simulink model "sm_suspension_templates"  (R2021b)
settings: Solver=ode15s  StartTime=0.0  StopTime=60  MaxStep=0.01  RelTol=1e-3  EnableMultiTasking=on
model workspace: external: MATLAB File sm_suspension_templates_params.m (data not in the file)
undefined symbols (not defined in the file or in its folder): dwb, mp, platform, pr, sm_suspension_templates_roadgen, wheel, X, Y, Z
libraries: sm_lib x108, sm_suspension_templates_lib x60, nesl_utility x7
(part 1 of 7)
CloseFcn:
  | clear simlog_sm_suspension_templates
Description:
  | Independent Suspension System Templates
settings Model: Creator=The MathWorks, Inc.  LastModifiedBy=The MathWorks, Inc.
settings SolverCC: AlgebraicLoopSolver=TrustRegion
settings DataIOCC: SaveFormat=Array  SaveOutput=off  ReturnWorkspaceOutputs=off
settings OptimizationCC: ExpressionDepthLimit=2147483647  LifeSpan=inf
settings DebuggingCC: UnderspecifiedInitializationDetection=Classic  MergeDetectMultiDrivingBlocksExec=none  AllowSymbolicDim=off  StateNameClashWarn=warning  SFUnexpectedBacktrackingDiag=warning  SFNoUnconditionalDefaultTransitionDiag=warning  SFExecutionAtInitializationDiag=none  SFMachineParentedDataDiag=warning  ArithmeticOperatorsInVariantConditions=warning
settings HardwareCC: ProdBitPerPointer=32  ProdBitPerSizeT=32  ProdBitPerPtrDiffT=32  ProdLargestAtomicFloat=None  ProdIntDivRoundTo=Undefined  ProdEndianess=Unspecified  ProdWordSize=32  ProdHWDeviceType=32-bit Generic
settings ModelReferenceCC: PropagateSignalLabelsOutOfModel=off
settings SFSimCC: SimUseLocalCustomCode=off  CustomCodeUndefinedFunction=UseInterfaceOnly
settings RTWCC: RTWUseLocalCustomCode=off
settings CodeAppCC: StateflowObjectComments=on
settings GRTTargetCC: TargetLangStandard=C89/C90 (ANSI)
settings ConfigComp: CovScope=ReferencedModels  CovIncludeTopModel=off  CovMetricSettings=dw  CovSaveCumulativeToWorkspaceVar=on  CovSaveSingleToWorkspaceVar=on  CovExternalEMLEnable=off  CovSFcnEnable=off
settings SimscapeCC: SimscapeNormalizeSystem=off  SimscapeNominalValues="[{\"value\":\"10\",\"unit\":\"V\"},{\"value\":\"1\",\"unit\":\"A\"},{\"value\":\"10\",\"unit\":\"N*m\"},{\"value\":\"10\",\"unit\":\"bar\"},{\"value\":\"100\",\"unit\":\"kJ/kg\"},{\"value\":\"1\",\"unit\":\"kW\"},{\"value\":\"300\",\"unit\":\"K\"},{\"value\":\"100\",\"unit\":\"cm^3/s\"},{\"value\":\"1\",\"unit\":\"kN\"},{\"value\":\"1\",\"unit\":\"g/cm^3\"},{\"value\":\"1\",\"unit\":\"l\"},{\"value\":\"1\",\"unit\":\"cm^2\"},{\"value\":\"60\",\"unit\":\"Hz\"}]"  SimscapeLogType=all  SimscapeLogSimulationStatistics=on  SimscapeLogName=simlog_sm_suspension_templates  SimscapeLogDataHistory=10000
settings ConfigurationSet: Description=SimMechanics 2G
settings DiagnosticsConfigSet: SimMechanicsUnconnectedFramePorts=none  SimMechanicsUnsatisfiedHighPriorityTargets=none
settings ExplorerConfigSet: InternalSimMechanicsExplorerSettings="<ExplorerConfiguration><canonicalview>default</canonicalview><AnimationSetting><BasePlaybackSpeed>1.0</BasePlaybackSpeed><PlaybackSpeedFactor>1.0</PlaybackSpeedFactor></AnimationSetting><TilePanel><TileInfo><Tiles Columns=\"1\" Count=\"1\" Rows=\"1\"><Column Left=\"2\" Weight=\"1\"/><Column Left=\"827\"/><Row Top=\"2\" Weight=\"1\"/><Row Top=\"666\"/><Tile Height=\"1\" Width=\"1\" X=\"0\" Y=\"0\"/></Tiles></TileInfo><SceneInfo><SceneViewer><BGColor><R>0.60000002384185791</R><G>0.60000002384185791</G><B>0.60000002384185791</B></BGColor><Camera><Position><X>0</X><Y>-4.48140033882927202</Y><Z>0.554502487182617188</Z></Position><Center><X>0</X><Y>-0.245328903198242188</Y><Z>0.554502487182617188</Z></Center><Up><X>0</X><Y>-0</Y><Z>1</Z></Up><Left>-1.15500002503395094</Left><Right>1.15500002503395094</Right><Bottom>-0.792227599024772688</Bottom><Top>0.792227599024772688</Top></Camera></SceneViewer></SceneInfo></TilePanel></ExplorerConfiguration>"

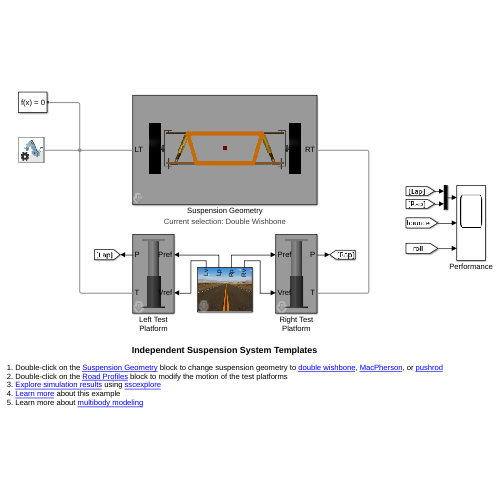
[thumbnail: Simulink's stored preview of the top-level diagram]
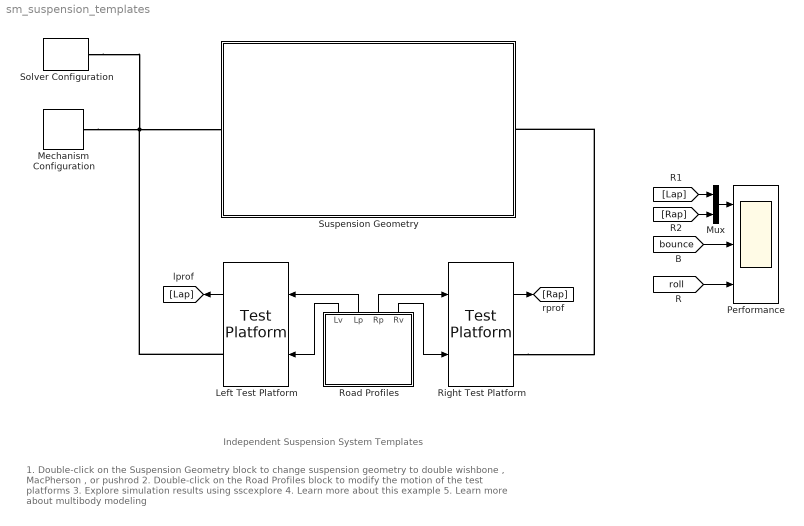
== system sm_suspension_templates ==
  note: Independent Suspension System Templates
  note: 1. Double-click on the Suspension Geometry block to change suspension geometry to double wishbone , MacPherson , or pushrod
      | 2. Double-click on the Road Profiles block to modify the motion of the test platforms
      | 3. Explore simulation results using sscexplore
      | 4. Learn more about this example
      | 5. Learn more about multibody modeling
  Left Test Platform : sm_suspension_templates_lib/Test Platform  Ro=platform.cylinder.outerradius  Ri=platform.cylinder.innerradius  Rf=platform.cylinder.flangeradius  Tf=platform.cylinder.flangethickness  Hc=platform.cylinder.height  cclr=platform.cylinder.color  loc=platform.cylinder.leftlocation  Rip=platform.piston.innerradius  Hp=platform.piston.height  pclr=platform.piston.color  L=platform.base.length  W=platform.base.width  H=platform.base.thickness  clr=platform.base.color  Kp=platform.controller.k  Kd=platform.controller.kd  rho=platform.density
      settings: SourceProductBaseCode=MS
  Mechanism Configuration : sm_lib/Utilities/Mechanism Configuration  UniformGravity=Constant  GravityVector=[0 0 -9.80665]  GravityUnits=m/s^2  LinearizationDelta=0.001  JointModeTransitionNonlinearIterations=2
  Mux : Mux  Inputs=2
  Performance : Scope  NumInputPorts=3
  Right Test Platform : sm_suspension_templates_lib/Test Platform  Ro=platform.cylinder.outerradius  Ri=platform.cylinder.innerradius  Rf=platform.cylinder.flangeradius  Tf=platform.cylinder.flangethickness  Hc=platform.cylinder.height  cclr=platform.cylinder.color  loc=platform.cylinder.rightlocation  Rip=platform.piston.innerradius  Hp=platform.piston.height  pclr=platform.piston.color  L=platform.base.length  W=platform.base.width  H=platform.base.thickness  clr=platform.base.color  Kp=platform.controller.k  Kd=platform.controller.kd  rho=platform.density
      settings: SourceProductBaseCode=MS
  Road Profiles : Subsystem  mask(Road Profile Generator){Ti=1, Ts=5.5, Tb=1, Fl=0.5, Al=5, Fm=3, Am=5, Fh=5, Ah=5, Ps=2, As=5, Wp=0.1, Pp=2, Ap=5, Ad=25}
      mask prompts: Ti "Start time (s):"; Ts "Duration of each segment (s):"; Tb "Buffer between segments (s):"; Fl "Frequency (Hz):"; Al "Amplitude (cm):"; Fm "Frequency (Hz):"; Am "Amplitude (cm):"; Fh "Frequency (Hz):"; Ah "Amplitude (cm):"; Ps "Period (s):"; As "Amplitude (cm):"; Wp "Width (s):"; Pp "Period (s):"; Ap "Amplitude (cm):"; Ad "Depth (cm):"
      mask help:
      | This block generates test road profiles for the left and right tires. A road profile is comprised of the following:
      |
      | 1  - Low frequency sinusoid with the left and right road profiles in phase
      | 2  - Low frequency sinusoid with the left and right road profiles out of phase
      | 3  - Mid frequency sinusoid with the left and right road profiles in phase
      | 4  - Mid frequency sinusoid with the left and right road profiles out of phase
      | 5  - High frequency sinusoid with the left and right road profiles in phase
      | 6  - High frequency sinusoid with the left and right road profiles out of phase
      | 7  - Step with the left and right road profiles in phase
      | 8  - Step with the left and right road profiles out of phase
      | 9  - Pulse with the left and right road profiles in phase
      | 10 - Pulse with the left and right road profiles out of phase
      | 11 - Large step down (dive)
      mask DialogControl ParameterTabVar0 Prompt: Time
      mask DialogControl ParameterTabVar01 Prompt: Low Freq
      mask DialogControl ParameterTabVar012 Prompt: Mid Freq
      mask DialogControl ParameterTabVar0123 Prompt: High Freq
      mask DialogControl ParameterTabVar01234 Prompt: Step
      mask DialogControl ParameterTabVar012345 Prompt: Pulse
      mask DialogControl ParameterTabVar0123456 Prompt: Dive
      mask Display:
      | image(imread(fullfile(matlabroot,...
      |     'toolbox','physmod','sm','smdemos',...
      |     'suspension_templates','images','sm_isuspension_road.png')));
  Solver Configuration : nesl_utility/Solver Configuration  PhysicalDomain=network_engine_domain  SubClassName=solver  LeftPortType=input  RightPortType=generic  Tones=[]  Harmonics=[]  SimulateNoise=off  Profile=off  UseLocalSampling=off  EnableSwitchedLinearOptims=on  FrequencyDomain=off  UseCCode=off  RelTol=0.001  AbsTol=1e-06  MinStep=1e-09  ToWorkspace=off  RevertToSquareIcSolve=off  NumHomotopyIterations=100  PhasorMode=off  PhasorModeNumHarmonics=1  DoDC=off  ResidualTolerance=1e-09  UseLocalSolver=off  LocalSolverChoice=NE_BACKWARD_EULER_ADVANCER  LocalSolverSampleTime=0.001  DoFixedCost=off  MaxNonlinIter=3  MaxModeIter=2  ComputeImpulses=off  ImpulseIterations=2  LinearAlgebra=Sparse  EquationFormulation=NE_TIME_EF  DelaysMemoryBudget=1024  AutomaticFiltering=on  FilteringTimeConstant=0.001  PartitionStorageMethod=AS_NEEDED  PartitionMemoryBudget=1024  PartitionMethod=FAST
      settings: SourceProductBaseCode=PW,SS
  Suspension Geometry : Subsystem  mask{SuspensionType=Double Wishbone}
      mask prompts: SuspensionType "Suspension Type:"
      mask init:
      | ST = get_param(gcb,'SuspensionType');
      | mdl = gcs;
      | switch ST
      |     case 'Double Wishbone'
      |         set_param([mdl,'/Suspension Geometry/Independent Suspension Geometry'],'OverrideUsingVariant','DoubleWishbone')
      |     case 'MacPherson'
      |         set_param([mdl,'/Suspension Geometry/Independent Suspension Geometry'],'OverrideUsingVariant','MacPherson')
      |     case 'Pushrod'
      |         set_param([mdl,'/Suspension Geometry/Independent Suspension Geometry'],'OverrideUsingVariant','Pushrod')
      | end
      settings: AttributesFormatString=Current selection: %<SuspensionType>
      mask TypeOptions SuspensionType: Double Wishbone | MacPherson | Pushrod
      mask Display:
      | ST = get_param(gcb,'SuspensionType');
      | switch ST
      |     case 'Double Wishbone'
      |         image(imread(fullfile(matlabroot,...
      |             'toolbox','physmod','sm','smdemos',...
      |             'suspension_templates','images','sm_isuspension_dwishboneassm.png')));
      |     case 'MacPherson'
      |         image(imread(fullfile(matlabroot,...
      |             'toolbox','physmod','sm','smdemos',...
      |             'suspension_templates','images','sm_isuspension_macphersonassm.png')));
      |     case 'Pushrod'
      |         image(imread(fullfile(matlabroot,...
      |             'toolbox','physmod','sm','smdemos',...
      |             'suspension_templates','images','sm_isuspension_pushrodassm.png')));
      | end
      | 
      | port_label('LConn',1,'LT');
      | port_label('RConn',1,'RT');
  wires:
  [bounce] -> Performance/2
  [roll] -> Performance/3
  [Lap] -> Mux/1
  [Rap] -> Mux/2
  Road Profiles/2(Lp) -> Left Test Platform/1
  Road Profiles/1(Lv) -> Left Test Platform/2
  Left Test Platform/1 -> [Lap]
  Right Test Platform/1 -> [Rap]
  Road Profiles/3(Rp) -> Right Test Platform/1
  Road Profiles/4(Rv) -> Right Test Platform/2
  Mux/1 -> Performance/1
  connections:
  Left Test Platform/RConn1 -- Suspension Geometry/LConn1 -- Solver Configuration/RConn1 -- Mechanism Configuration/RConn1
  Right Test Platform/RConn1 -- Suspension Geometry/RConn1

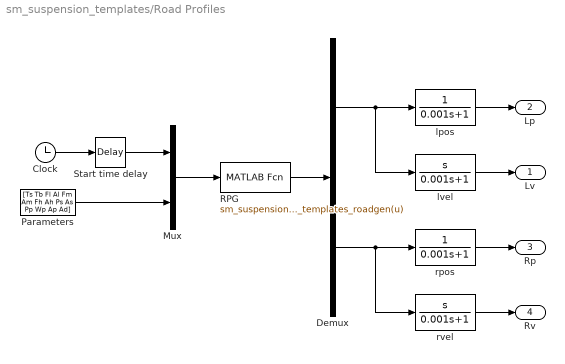
== system sm_suspension_templates/Road Profiles ==
  Clock : Clock
  Demux : Demux  Outputs=2
  Mux : Mux  Inputs=2
  Parameters : Constant  Value=[Ts Tb Fl Al Fm Am Fh Ah Ps As Pp Wp Ap Ad]
  RPG : MATLABFcn  MATLABFcn=sm_suspension_templates_roadgen(u)  Output1D=off
  Start time delay : TransportDelay  DelayTime=Ti  BufferSize=2048
  lpos : TransferFcn  Denominator=[0.001 1]
  lvel : TransferFcn  Numerator=[1 0]  Denominator=[0.001 1]
  rpos : TransferFcn  Denominator=[0.001 1]
  rvel : TransferFcn  Numerator=[1 0]  Denominator=[0.001 1]
  Lv : Outport  VectorParamsAs1DForOutWhenUnconnected=off
  Lp : Outport  Port=2  VectorParamsAs1DForOutWhenUnconnected=off
  Rp : Outport  Port=3  VectorParamsAs1DForOutWhenUnconnected=off
  Rv : Outport  Port=4  VectorParamsAs1DForOutWhenUnconnected=off
  wires:
  Demux/1 -> lpos/1, lvel/1
  lpos/1 -> Lp/1
  lvel/1 -> Lv/1
  Demux/2 -> rvel/1, rpos/1
  rpos/1 -> Rp/1
  rvel/1 -> Rv/1
  Clock/1 -> Start time delay/1
  Parameters/1 -> Mux/2
  Mux/1 -> RPG/1
  RPG/1 -> Demux/1
  Start time delay/1 -> Mux/1

== system sm_suspension_templates/Suspension Geometry ==
  Independent Suspension Geometry : Subsystem  BlockChoice=MacPherson  Variant=on  VariantControlMode=label  LabelModeActiveChoice=DoubleWishbone
      settings: AttributesFormatString=%<ActiveVariant>
      mask Display:
      | ST = get_param(gcb,'ActiveVariant');
      | switch ST
      |     case 'DoubleWishbone'
      |         image(imread(fullfile(matlabroot,...
      |             'toolbox','physmod','sm','smdemos',...
      |             'suspension_templates','images','sm_isuspension_dwishbone.png')));
      |     case 'MacPherson'
      |         image(imread(fullfile(matlabroot,...
      |             'toolbox','physmod','sm','smdemos',...
      |             'suspension_templates','images','sm_isuspension_macpherson.png')));
      |     case 'Pushrod'
      |         image(imread(fullfile(matlabroot,...
      |             'toolbox','physmod','sm','smdemos',...
      |             'suspension_templates','images','sm_isuspension_pushrod.png')));
      | end
  Rigid Transform : sm_lib/Frames and Transforms/Rigid Transform  TranslationMethod=None  TranslationStandardOffset=0  TranslationLengthUnit=m  TranslationStandardAxis=+Z  TranslationCartesianOffset=[0 0 0]  TranslationROffset=0  TranslationROffsetUnits=m  TranslationZOffset=0  TranslationZOffsetUnits=m  TranslationThetaOffset=0  TranslationThetaOffsetUnits=deg  RotationMethod=AlignedAxes  RotationAngleUnits=deg  RotationStandardAxis=+Z  RotationAngle=0  RotationArbitraryAxis=[0 0 1]  FollAlignAxisA=+X  BaseAlignAxisA=-X  FollAlignAxisB=+Z  BaseAlignAxisB=+Z  RotationSequenceAxes=FollowerAxes  RotationSequence=XYX  RotationSequenceAngles=[0 0 0]  RotationSequenceAnglesUnits=deg  RotationMatrix=[1 0 0; 0 1 0; 0 0 1]
  Wheel L : sm_suspension_templates_lib/Wheel  Rti=wheel.tire.innerradius  Rto=wheel.tire.outerradius  Wt=wheel.tire.width  Rtr=wheel.tire.chamferradius  trho=wheel.tire.density  tclr=wheel.tire.color  Rhi=wheel.hub.radius  Rho=wheel.hub.outerradius  Ns=wheel.hub.numspokes  Ts=wheel.hub.spokethickness  Wh=wheel.hub.width  srho=wheel.hub.density  sclr=wheel.hub.color  Ls=wheel.shaft.length  Rs=wheel.shaft.radius  Rb=wheel.disc.radius  Tb=wheel.disc.thickness
      settings: SourceProductBaseCode=MS
  Wheel R : sm_suspension_templates_lib/Wheel  Rti=wheel.tire.innerradius  Rto=wheel.tire.outerradius  Wt=wheel.tire.width  Rtr=wheel.tire.chamferradius  trho=wheel.tire.density  tclr=wheel.tire.color  Rhi=wheel.hub.radius  Rho=wheel.hub.outerradius  Ns=wheel.hub.numspokes  Ts=wheel.hub.spokethickness  Wh=wheel.hub.width  srho=wheel.hub.density  sclr=wheel.hub.color  Ls=wheel.shaft.length  Rs=wheel.shaft.radius  Rb=wheel.disc.radius  Tb=wheel.disc.thickness
      settings: SourceProductBaseCode=MS
  LT : PMIOPort  Side=Left
  RT : PMIOPort  Port=2  Side=Right
  connections:
  Rigid Transform/RConn1 -- LT/RConn1
  Wheel L/RConn1 -- Rigid Transform/LConn1
  Wheel R/RConn1 -- RT/RConn1
  Independent Suspension Geometry/LConn1 -- Wheel L/LConn1
  Independent Suspension Geometry/RConn1 -- Wheel R/LConn1

== system sm_suspension_templates/Suspension Geometry/Independent Suspension Geometry ==
  Double Wishbone : Subsystem  VariantControl=DoubleWishbone
      mask Display:
      | image(imread(fullfile(matlabroot,...
      |     'toolbox','physmod','sm','smdemos',...
      |     'suspension_templates','images','sm_isuspension_dwishbone.png')));
  MacPherson : Subsystem  VariantControl=MacPherson
      mask Display:
      | image(imread(fullfile(matlabroot,...
      |     'toolbox','physmod','sm','smdemos',...
      |     'suspension_templates','images','sm_isuspension_macpherson.png')));
  Pushrod : Subsystem  VariantControl=Pushrod
      mask Display:
      | image(imread(fullfile(matlabroot,...
      |     'toolbox','physmod','sm','smdemos',...
      |     'suspension_templates','images','sm_isuspension_pushrod.png')));
  L_Wheel_Axle : PMIOPort  Side=Left
  R_Wheel_Axle : PMIOPort  Port=2  Side=Right

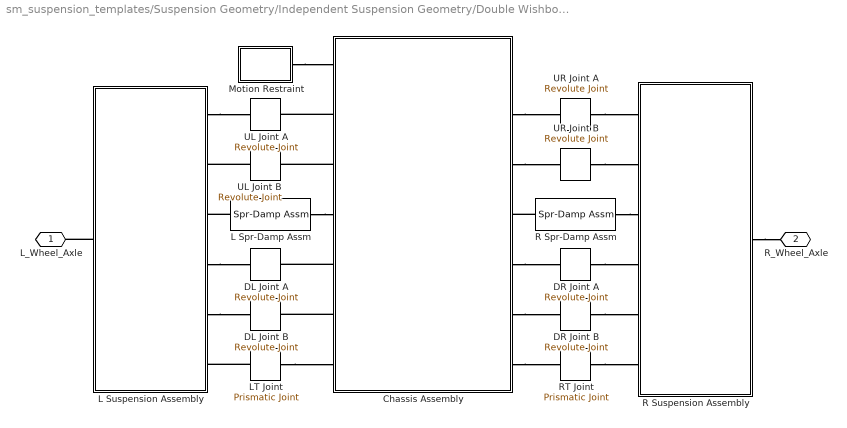
== system sm_suspension_templates/Suspension Geometry/Independent Suspension Geometry/Double Wishbone ==
  Chassis Assembly : Subsystem
      mask Display:
      | image(imread(fullfile(matlabroot,...
      |     'toolbox','physmod','sm','smdemos',...
      |     'suspension_templates','images','sm_isuspension_frameassm.png')));
      | 
      | port_label('LConn',1,'BC');
      | port_label('LConn',2,'ULA');
      | port_label('LConn',3,'ULB');
      | port_label('LConn',4,'ULC');
      | port_label('LConn',5,'DLA');
      | port_label('LConn',6,'DLB');
      | port_label('LConn',7,'LT');
      | port_label('RConn',1,'FC');
      | port_label('RConn',2,'URA');
      | port_label('RConn',3,'URB');
      | port_label('RConn',4,'URC');
      | port_label('RConn',5,'DRA');
      | port_label('RConn',6,'DRB');
      | port_label('RConn',7,'RT');
  DL Joint A : sm_lib/Joints/Revolute Joint  JointMode=Normal  SenseConstraintForce=off  SenseConstraintForceX=off  SenseConstraintForceY=off  SenseConstraintForceZ=off  SenseConstraintTorque=off  SenseConstraintTorqueX=off  SenseConstraintTorqueY=off  SenseConstraintTorqueZ=off  SenseTotalForce=off  SenseTotalForceX=off  SenseTotalForceY=off  SenseTotalForceZ=off  SenseTotalTorque=off  SenseTotalTorqueX=off  SenseTotalTorqueY=off  SenseTotalTorqueZ=off  CompositeWrenchDir=FollowerOnBase  CompositeWrenchFrame=BaseFrame  EquilibriumPosition=0  EquilibriumPositionUnits=deg  SpringStiffness=0  SpringStiffnessUnits=N*m/deg  DampingCoefficient=0  DampingCoefficientUnits=N*m/(deg/s)  TorqueActuationMode=NoTorque  MotionActuationMode=ComputedMotion  SensePosition=off  SenseVelocity=off  SenseAcceleration=off  SenseTorqueForce=off  SenseLowerLimitTorqueForce=off  SenseUpperLimitTorqueForce=off  LowerLimitSpecify=off  LowerLimitBound=-90  LowerLimitBoundUnits=deg  LowerLimitStiffness=1e4  LowerLimitStiffnessUnits=N*m/deg  LowerLimitDamping=10  LowerLimitDampingUnits=N*m/(deg/s)  LowerLimitTransitionRegionWidth=0.1  LowerLimitTransitionRegionWidthUnits=deg  UpperLimitSpecify=off  UpperLimitBound=90  UpperLimitBoundUnits=deg  UpperLimitStiffness=1e4  UpperLimitStiffnessUnits=N*m/deg  UpperLimitDamping=10  UpperLimitDampingUnits=N*m/(deg/s)  UpperLimitTransitionRegionWidth=0.1  UpperLimitTransitionRegionWidthUnits=deg  PositionTargetSpecify=on  PositionTargetPriority=High  PositionTargetValue=0  PositionTargetValueUnits=deg  VelocityTargetSpecify=off  VelocityTargetPriority=High  VelocityTargetValue=0  VelocityTargetValueUnits=deg/s
  DL Joint B : sm_lib/Joints/Revolute Joint  JointMode=Normal  SenseConstraintForce=off  SenseConstraintForceX=off  SenseConstraintForceY=off  SenseConstraintForceZ=off  SenseConstraintTorque=off  SenseConstraintTorqueX=off  SenseConstraintTorqueY=off  SenseConstraintTorqueZ=off  SenseTotalForce=off  SenseTotalForceX=off  SenseTotalForceY=off  SenseTotalForceZ=off  SenseTotalTorque=off  SenseTotalTorqueX=off  SenseTotalTorqueY=off  SenseTotalTorqueZ=off  CompositeWrenchDir=FollowerOnBase  CompositeWrenchFrame=BaseFrame  EquilibriumPosition=0  EquilibriumPositionUnits=deg  SpringStiffness=0  SpringStiffnessUnits=N*m/deg  DampingCoefficient=0  DampingCoefficientUnits=N*m/(deg/s)  TorqueActuationMode=NoTorque  MotionActuationMode=ComputedMotion  SensePosition=off  SenseVelocity=off  SenseAcceleration=off  SenseTorqueForce=off  SenseLowerLimitTorqueForce=off  SenseUpperLimitTorqueForce=off  LowerLimitSpecify=off  LowerLimitBound=-90  LowerLimitBoundUnits=deg  LowerLimitStiffness=1e4  LowerLimitStiffnessUnits=N*m/deg  LowerLimitDamping=10  LowerLimitDampingUnits=N*m/(deg/s)  LowerLimitTransitionRegionWidth=0.1  LowerLimitTransitionRegionWidthUnits=deg  UpperLimitSpecify=off  UpperLimitBound=90  UpperLimitBoundUnits=deg  UpperLimitStiffness=1e4  UpperLimitStiffnessUnits=N*m/deg  UpperLimitDamping=10  UpperLimitDampingUnits=N*m/(deg/s)  UpperLimitTransitionRegionWidth=0.1  UpperLimitTransitionRegionWidthUnits=deg  PositionTargetSpecify=off  PositionTargetPriority=High  PositionTargetValue=90  PositionTargetValueUnits=deg  VelocityTargetSpecify=off  VelocityTargetPriority=High  VelocityTargetValue=0  VelocityTargetValueUnits=deg/s
  DR Joint A : sm_lib/Joints/Revolute Joint  JointMode=Normal  SenseConstraintForce=off  SenseConstraintForceX=off  SenseConstraintForceY=off  SenseConstraintForceZ=off  SenseConstraintTorque=off  SenseConstraintTorqueX=off  SenseConstraintTorqueY=off  SenseConstraintTorqueZ=off  SenseTotalForce=off  SenseTotalForceX=off  SenseTotalForceY=off  SenseTotalForceZ=off  SenseTotalTorque=off  SenseTotalTorqueX=off  SenseTotalTorqueY=off  SenseTotalTorqueZ=off  CompositeWrenchDir=FollowerOnBase  CompositeWrenchFrame=BaseFrame  EquilibriumPosition=0  EquilibriumPositionUnits=deg  SpringStiffness=0  SpringStiffnessUnits=N*m/deg  DampingCoefficient=0  DampingCoefficientUnits=N*m/(deg/s)  TorqueActuationMode=NoTorque  MotionActuationMode=ComputedMotion  SensePosition=off  SenseVelocity=off  SenseAcceleration=off  SenseTorqueForce=off  SenseLowerLimitTorqueForce=off  SenseUpperLimitTorqueForce=off  LowerLimitSpecify=off  LowerLimitBound=-90  LowerLimitBoundUnits=deg  LowerLimitStiffness=1e4  LowerLimitStiffnessUnits=N*m/deg  LowerLimitDamping=10  LowerLimitDampingUnits=N*m/(deg/s)  LowerLimitTransitionRegionWidth=0.1  LowerLimitTransitionRegionWidthUnits=deg  UpperLimitSpecify=off  UpperLimitBound=90  UpperLimitBoundUnits=deg  UpperLimitStiffness=1e4  UpperLimitStiffnessUnits=N*m/deg  UpperLimitDamping=10  UpperLimitDampingUnits=N*m/(deg/s)  UpperLimitTransitionRegionWidth=0.1  UpperLimitTransitionRegionWidthUnits=deg  PositionTargetSpecify=on  PositionTargetPriority=High  PositionTargetValue=0  PositionTargetValueUnits=deg  VelocityTargetSpecify=off  VelocityTargetPriority=High  VelocityTargetValue=0  VelocityTargetValueUnits=deg/s
  DR Joint B : sm_lib/Joints/Revolute Joint  JointMode=Normal  SenseConstraintForce=off  SenseConstraintForceX=off  SenseConstraintForceY=off  SenseConstraintForceZ=off  SenseConstraintTorque=off  SenseConstraintTorqueX=off  SenseConstraintTorqueY=off  SenseConstraintTorqueZ=off  SenseTotalForce=off  SenseTotalForceX=off  SenseTotalForceY=off  SenseTotalForceZ=off  SenseTotalTorque=off  SenseTotalTorqueX=off  SenseTotalTorqueY=off  SenseTotalTorqueZ=off  CompositeWrenchDir=FollowerOnBase  CompositeWrenchFrame=BaseFrame  EquilibriumPosition=0  EquilibriumPositionUnits=deg  SpringStiffness=0  SpringStiffnessUnits=N*m/deg  DampingCoefficient=0  DampingCoefficientUnits=N*m/(deg/s)  TorqueActuationMode=NoTorque  MotionActuationMode=ComputedMotion  SensePosition=off  SenseVelocity=off  SenseAcceleration=off  SenseTorqueForce=off  SenseLowerLimitTorqueForce=off  SenseUpperLimitTorqueForce=off  LowerLimitSpecify=off  LowerLimitBound=-90  LowerLimitBoundUnits=deg  LowerLimitStiffness=1e4  LowerLimitStiffnessUnits=N*m/deg  LowerLimitDamping=10  LowerLimitDampingUnits=N*m/(deg/s)  LowerLimitTransitionRegionWidth=0.1  LowerLimitTransitionRegionWidthUnits=deg  UpperLimitSpecify=off  UpperLimitBound=90  UpperLimitBoundUnits=deg  UpperLimitStiffness=1e4  UpperLimitStiffnessUnits=N*m/deg  UpperLimitDamping=10  UpperLimitDampingUnits=N*m/(deg/s)  UpperLimitTransitionRegionWidth=0.1  UpperLimitTransitionRegionWidthUnits=deg  PositionTargetSpecify=off  PositionTargetPriority=High  PositionTargetValue=90  PositionTargetValueUnits=deg  VelocityTargetSpecify=off  VelocityTargetPriority=High  VelocityTargetValue=0  VelocityTargetValueUnits=deg/s
  L Spr-Damp Assm : sm_suspension_templates_lib/Spr-Damp Assm  Ks=dwb.springdamp.k  Kb=dwb.springdamp.b  Ls=dwb.springdamp.length0  Lc=dwb.springdamp.cylinder.length  Rci=dwb.springdamp.cylinder.innerradius  Rco=dwb.springdamp.cylinder.outerradius  Lp=dwb.springdamp.piston.length  Rr=dwb.springdamp.chamferradius  Lb=dwb.springdamp.bracket.length  Wb=dwb.springdamp.bracket.width  Tb=dwb.springdamp.bracket.thickness  Rbh=dwb.springdamp.bracket.holeradius  rho=dwb.springdamp.density  cclr=dwb.springdamp.cylinder.color  pclr=dwb.springdamp.piston.color
      settings: SourceProductBaseCode=MS
  L Suspension Assembly : Subsystem
      mask Display:
      | image(imread(fullfile(matlabroot,...
      |     'toolbox','physmod','sm','smdemos',...
      |     'suspension_templates','images','sm_isuspension_dwishbonesuspensionassm.png')));
      | 
      | port_label('LConn',1,'W');
      | port_label('RConn',1,'UA');
      | port_label('RConn',2,'UB');
      | port_label('RConn',3,'DP');
      | port_label('RConn',4,'DA');
      | port_label('RConn',5,'DB');
      | port_label('RConn',6,'LT');
  LT Joint : sm_lib/Joints/Prismatic Joint  JointMode=Normal  SenseConstraintForce=off  SenseConstraintForceX=off  SenseConstraintForceY=off  SenseConstraintForceZ=off  SenseConstraintTorque=off  SenseConstraintTorqueX=off  SenseConstraintTorqueY=off  SenseConstraintTorqueZ=off  SenseTotalForce=off  SenseTotalForceX=off  SenseTotalForceY=off  SenseTotalForceZ=off  SenseTotalTorque=off  SenseTotalTorqueX=off  SenseTotalTorqueY=off  SenseTotalTorqueZ=off  CompositeWrenchDir=FollowerOnBase  CompositeWrenchFrame=BaseFrame  EquilibriumPosition=0  EquilibriumPositionUnits=m  SpringStiffness=0  SpringStiffnessUnits=N/m  DampingCoefficient=0  DampingCoefficientUnits=N/(m/s)  TorqueActuationMode=NoTorque  MotionActuationMode=ComputedMotion  SensePosition=off  SenseVelocity=off  SenseAcceleration=off  SenseTorqueForce=off  SenseLowerLimitTorqueForce=off  SenseUpperLimitTorqueForce=off  LowerLimitSpecify=off  LowerLimitBound=-1  LowerLimitBoundUnits=m  LowerLimitStiffness=1e6  LowerLimitStiffnessUnits=N/m  LowerLimitDamping=1e3  LowerLimitDampingUnits=N/(m/s)  LowerLimitTransitionRegionWidth=1e-4  LowerLimitTransitionRegionWidthUnits=m  UpperLimitSpecify=off  UpperLimitBound=1  UpperLimitBoundUnits=m  UpperLimitStiffness=1e6  UpperLimitStiffnessUnits=N/m  UpperLimitDamping=1e3  UpperLimitDampingUnits=N/(m/s)  UpperLimitTransitionRegionWidth=1e-4  UpperLimitTransitionRegionWidthUnits=m  PositionTargetSpecify=off  PositionTargetPriority=High  PositionTargetValue=0  PositionTargetValueUnits=m  VelocityTargetSpecify=off  VelocityTargetPriority=High  VelocityTargetValue=0  VelocityTargetValueUnits=m/s
  Motion Restraint : Subsystem
  R Spr-Damp Assm : sm_suspension_templates_lib/Spr-Damp Assm  Ks=dwb.springdamp.k  Kb=dwb.springdamp.b  Ls=dwb.springdamp.length0  Lc=dwb.springdamp.cylinder.length  Rci=dwb.springdamp.cylinder.innerradius  Rco=dwb.springdamp.cylinder.outerradius  Lp=dwb.springdamp.piston.length  Rr=dwb.springdamp.chamferradius  Lb=dwb.springdamp.bracket.length  Wb=dwb.springdamp.bracket.width  Tb=dwb.springdamp.bracket.thickness  Rbh=dwb.springdamp.bracket.holeradius  rho=dwb.springdamp.density  cclr=dwb.springdamp.cylinder.color  pclr=dwb.springdamp.piston.color
      settings: SourceProductBaseCode=MS
  R Suspension Assembly : Subsystem
      mask Display:
      | image(imread(fullfile(matlabroot,...
      |     'toolbox','physmod','sm','smdemos',...
      |     'suspension_templates','images','sm_isuspension_dwishbonesuspensionassm.png')));
      | 
      | port_label('RConn',1,'T');
      | port_label('LConn',1,'UA');
      | port_label('LConn',2,'UB');
      | port_label('LConn',3,'DP');
      | port_label('LConn',4,'DA');
      | port_label('LConn',5,'DB');
      | port_label('LConn',6,'RT');
  RT Joint : sm_lib/Joints/Prismatic Joint  JointMode=Normal  SenseConstraintForce=off  SenseConstraintForceX=off  SenseConstraintForceY=off  SenseConstraintForceZ=off  SenseConstraintTorque=off  SenseConstraintTorqueX=off  SenseConstraintTorqueY=off  SenseConstraintTorqueZ=off  SenseTotalForce=off  SenseTotalForceX=off  SenseTotalForceY=off  SenseTotalForceZ=off  SenseTotalTorque=off  SenseTotalTorqueX=off  SenseTotalTorqueY=off  SenseTotalTorqueZ=off  CompositeWrenchDir=FollowerOnBase  CompositeWrenchFrame=BaseFrame  EquilibriumPosition=0  EquilibriumPositionUnits=m  SpringStiffness=0  SpringStiffnessUnits=N/m  DampingCoefficient=0  DampingCoefficientUnits=N/(m/s)  TorqueActuationMode=NoTorque  MotionActuationMode=ComputedMotion  SensePosition=off  SenseVelocity=off  SenseAcceleration=off  SenseTorqueForce=off  SenseLowerLimitTorqueForce=off  SenseUpperLimitTorqueForce=off  LowerLimitSpecify=off  LowerLimitBound=-1  LowerLimitBoundUnits=m  LowerLimitStiffness=1e6  LowerLimitStiffnessUnits=N/m  LowerLimitDamping=1e3  LowerLimitDampingUnits=N/(m/s)  LowerLimitTransitionRegionWidth=1e-4  LowerLimitTransitionRegionWidthUnits=m  UpperLimitSpecify=off  UpperLimitBound=1  UpperLimitBoundUnits=m  UpperLimitStiffness=1e6  UpperLimitStiffnessUnits=N/m  UpperLimitDamping=1e3  UpperLimitDampingUnits=N/(m/s)  UpperLimitTransitionRegionWidth=1e-4  UpperLimitTransitionRegionWidthUnits=m  PositionTargetSpecify=off  PositionTargetPriority=High  PositionTargetValue=0  PositionTargetValueUnits=m  VelocityTargetSpecify=off  VelocityTargetPriority=High  VelocityTargetValue=0  VelocityTargetValueUnits=m/s
  UL Joint A : sm_lib/Joints/Revolute Joint  JointMode=Normal  SenseConstraintForce=off  SenseConstraintForceX=off  SenseConstraintForceY=off  SenseConstraintForceZ=off  SenseConstraintTorque=off  SenseConstraintTorqueX=off  SenseConstraintTorqueY=off  SenseConstraintTorqueZ=off  SenseTotalForce=off  SenseTotalForceX=off  SenseTotalForceY=off  SenseTotalForceZ=off  SenseTotalTorque=off  SenseTotalTorqueX=off  SenseTotalTorqueY=off  SenseTotalTorqueZ=off  CompositeWrenchDir=FollowerOnBase  CompositeWrenchFrame=BaseFrame  EquilibriumPosition=0  EquilibriumPositionUnits=deg  SpringStiffness=0  SpringStiffnessUnits=N*m/deg  DampingCoefficient=0  DampingCoefficientUnits=N*m/(deg/s)  TorqueActuationMode=NoTorque  MotionActuationMode=ComputedMotion  SensePosition=off  SenseVelocity=off  SenseAcceleration=off  SenseTorqueForce=off  SenseLowerLimitTorqueForce=off  SenseUpperLimitTorqueForce=off  LowerLimitSpecify=off  LowerLimitBound=-90  LowerLimitBoundUnits=deg  LowerLimitStiffness=1e4  LowerLimitStiffnessUnits=N*m/deg  LowerLimitDamping=10  LowerLimitDampingUnits=N*m/(deg/s)  LowerLimitTransitionRegionWidth=0.1  LowerLimitTransitionRegionWidthUnits=deg  UpperLimitSpecify=off  UpperLimitBound=90  UpperLimitBoundUnits=deg  UpperLimitStiffness=1e4  UpperLimitStiffnessUnits=N*m/deg  UpperLimitDamping=10  UpperLimitDampingUnits=N*m/(deg/s)  UpperLimitTransitionRegionWidth=0.1  UpperLimitTransitionRegionWidthUnits=deg  PositionTargetSpecify=off  PositionTargetPriority=Low  PositionTargetValue=180  PositionTargetValueUnits=deg  VelocityTargetSpecify=off  VelocityTargetPriority=High  VelocityTargetValue=0  VelocityTargetValueUnits=deg/s
  UL Joint B : sm_lib/Joints/Revolute Joint  JointMode=Normal  SenseConstraintForce=off  SenseConstraintForceX=off  SenseConstraintForceY=off  SenseConstraintForceZ=off  SenseConstraintTorque=off  SenseConstraintTorqueX=off  SenseConstraintTorqueY=off  SenseConstraintTorqueZ=off  SenseTotalForce=off  SenseTotalForceX=off  SenseTotalForceY=off  SenseTotalForceZ=off  SenseTotalTorque=off  SenseTotalTorqueX=off  SenseTotalTorqueY=off  SenseTotalTorqueZ=off  CompositeWrenchDir=FollowerOnBase  CompositeWrenchFrame=BaseFrame  EquilibriumPosition=0  EquilibriumPositionUnits=deg  SpringStiffness=0  SpringStiffnessUnits=N*m/deg  DampingCoefficient=0  DampingCoefficientUnits=N*m/(deg/s)  TorqueActuationMode=NoTorque  MotionActuationMode=ComputedMotion  SensePosition=off  SenseVelocity=off  SenseAcceleration=off  SenseTorqueForce=off  SenseLowerLimitTorqueForce=off  SenseUpperLimitTorqueForce=off  LowerLimitSpecify=off  LowerLimitBound=-90  LowerLimitBoundUnits=deg  LowerLimitStiffness=1e4  LowerLimitStiffnessUnits=N*m/deg  LowerLimitDamping=10  LowerLimitDampingUnits=N*m/(deg/s)  LowerLimitTransitionRegionWidth=0.1  LowerLimitTransitionRegionWidthUnits=deg  UpperLimitSpecify=off  UpperLimitBound=90  UpperLimitBoundUnits=deg  UpperLimitStiffness=1e4  UpperLimitStiffnessUnits=N*m/deg  UpperLimitDamping=10  UpperLimitDampingUnits=N*m/(deg/s)  UpperLimitTransitionRegionWidth=0.1  UpperLimitTransitionRegionWidthUnits=deg  PositionTargetSpecify=off  PositionTargetPriority=High  PositionTargetValue=90  PositionTargetValueUnits=deg  VelocityTargetSpecify=off  VelocityTargetPriority=High  VelocityTargetValue=0  VelocityTargetValueUnits=deg/s
  UR Joint A : sm_lib/Joints/Revolute Joint  JointMode=Normal  SenseConstraintForce=off  SenseConstraintForceX=off  SenseConstraintForceY=off  SenseConstraintForceZ=off  SenseConstraintTorque=off  SenseConstraintTorqueX=off  SenseConstraintTorqueY=off  SenseConstraintTorqueZ=off  SenseTotalForce=off  SenseTotalForceX=off  SenseTotalForceY=off  SenseTotalForceZ=off  SenseTotalTorque=off  SenseTotalTorqueX=off  SenseTotalTorqueY=off  SenseTotalTorqueZ=off  CompositeWrenchDir=FollowerOnBase  CompositeWrenchFrame=BaseFrame  EquilibriumPosition=0  EquilibriumPositionUnits=deg  SpringStiffness=0  SpringStiffnessUnits=N*m/deg  DampingCoefficient=0  DampingCoefficientUnits=N*m/(deg/s)  TorqueActuationMode=NoTorque  MotionActuationMode=ComputedMotion  SensePosition=off  SenseVelocity=off  SenseAcceleration=off  SenseTorqueForce=off  SenseLowerLimitTorqueForce=off  SenseUpperLimitTorqueForce=off  LowerLimitSpecify=off  LowerLimitBound=-90  LowerLimitBoundUnits=deg  LowerLimitStiffness=1e4  LowerLimitStiffnessUnits=N*m/deg  LowerLimitDamping=10  LowerLimitDampingUnits=N*m/(deg/s)  LowerLimitTransitionRegionWidth=0.1  LowerLimitTransitionRegionWidthUnits=deg  UpperLimitSpecify=off  UpperLimitBound=90  UpperLimitBoundUnits=deg  UpperLimitStiffness=1e4  UpperLimitStiffnessUnits=N*m/deg  UpperLimitDamping=10  UpperLimitDampingUnits=N*m/(deg/s)  UpperLimitTransitionRegionWidth=0.1  UpperLimitTransitionRegionWidthUnits=deg  PositionTargetSpecify=off  PositionTargetPriority=High  PositionTargetValue=90  PositionTargetValueUnits=deg  VelocityTargetSpecify=off  VelocityTargetPriority=High  VelocityTargetValue=0  VelocityTargetValueUnits=deg/s
  UR Joint B : sm_lib/Joints/Revolute Joint  JointMode=Normal  SenseConstraintForce=off  SenseConstraintForceX=off  SenseConstraintForceY=off  SenseConstraintForceZ=off  SenseConstraintTorque=off  SenseConstraintTorqueX=off  SenseConstraintTorqueY=off  SenseConstraintTorqueZ=off  SenseTotalForce=off  SenseTotalForceX=off  SenseTotalForceY=off  SenseTotalForceZ=off  SenseTotalTorque=off  SenseTotalTorqueX=off  SenseTotalTorqueY=off  SenseTotalTorqueZ=off  CompositeWrenchDir=FollowerOnBase  CompositeWrenchFrame=BaseFrame  EquilibriumPosition=0  EquilibriumPositionUnits=deg  SpringStiffness=0  SpringStiffnessUnits=N*m/deg  DampingCoefficient=0  DampingCoefficientUnits=N*m/(deg/s)  TorqueActuationMode=NoTorque  MotionActuationMode=ComputedMotion  SensePosition=off  SenseVelocity=off  SenseAcceleration=off  SenseTorqueForce=off  SenseLowerLimitTorqueForce=off  SenseUpperLimitTorqueForce=off  LowerLimitSpecify=off  LowerLimitBound=-90  LowerLimitBoundUnits=deg  LowerLimitStiffness=1e4  LowerLimitStiffnessUnits=N*m/deg  LowerLimitDamping=10  LowerLimitDampingUnits=N*m/(deg/s)  LowerLimitTransitionRegionWidth=0.1  LowerLimitTransitionRegionWidthUnits=deg  UpperLimitSpecify=off  UpperLimitBound=90  UpperLimitBoundUnits=deg  UpperLimitStiffness=1e4  UpperLimitStiffnessUnits=N*m/deg  UpperLimitDamping=10  UpperLimitDampingUnits=N*m/(deg/s)  UpperLimitTransitionRegionWidth=0.1  UpperLimitTransitionRegionWidthUnits=deg  PositionTargetSpecify=off  PositionTargetPriority=High  PositionTargetValue=0  PositionTargetValueUnits=deg  VelocityTargetSpecify=off  VelocityTargetPriority=High  VelocityTargetValue=0  VelocityTargetValueUnits=deg/s
  L_Wheel_Axle : PMIOPort  Side=Left
  R_Wheel_Axle : PMIOPort  Port=2  Side=Right
  connections:
  UR Joint A/RConn1 -- R Suspension Assembly/LConn1
  UR Joint B/RConn1 -- R Suspension Assembly/LConn2
  DR Joint A/RConn1 -- R Suspension Assembly/LConn4
  DR Joint B/RConn1 -- R Suspension Assembly/LConn5
  Chassis Assembly/RConn2 -- UR Joint A/LConn1
  Chassis Assembly/RConn3 -- UR Joint B/LConn1
  Chassis Assembly/RConn5 -- DR Joint A/LConn1
  Chassis Assembly/RConn6 -- DR Joint B/LConn1
  R Spr-Damp Assm/LConn1 -- Chassis Assembly/RConn4
  R Spr-Damp Assm/RConn1 -- R Suspension Assembly/LConn3
  Motion Restraint/RConn1 -- Chassis Assembly/LConn1
  Chassis Assembly/LConn6 -- DL Joint B/LConn1
  UL Joint B/RConn1 -- L Suspension Assembly/RConn2
  Chassis Assembly/LConn3 -- UL Joint B/LConn1
  L Suspension Assembly/RConn1 -- UL Joint A/RConn1
  L Suspension Assembly/RConn5 -- DL Joint B/RConn1
  L Suspension Assembly/RConn4 -- DL Joint A/RConn1
  Chassis Assembly/LConn5 -- DL Joint A/LConn1
  Chassis Assembly/LConn2 -- UL Joint A/LConn1
  L Spr-Damp Assm/LConn1 -- Chassis Assembly/LConn4
  Chassis Assembly/RConn7 -- RT Joint/LConn1
  L Spr-Damp Assm/RConn1 -- L Suspension Assembly/RConn3
  RT Joint/RConn1 -- R Suspension Assembly/LConn6
  LT Joint/LConn1 -- Chassis Assembly/LConn7
  LT Joint/RConn1 -- L Suspension Assembly/RConn6
  R Suspension Assembly/RConn1 -- R_Wheel_Axle/RConn1
  L Suspension Assembly/LConn1 -- L_Wheel_Axle/RConn1
